simulink model "SPGF_FSK_0000_R2019b"  (R2019b)
settings: Solver=ode3  SolverName=ode4  StartTime=0.0  StopTime=1.4  FixedStep=50e-6/50  RelTol=1e-3  EnableMultiTasking=on
undefined symbols (not defined in the file): D11, Delta
libraries: powerlib x2544, powerlib_meascontrol x204, simulink x24
(part 29 of 33)

== system SPGF_FSK_0000_R2019b/W60/Pi ==
  Ground{,1..8} (9 alike) : powerlib/Elements/Ground  LConnTagsString=a
  Series RLC Branch{,1..2,27..28,33} (6 alike) : powerlib/Elements/Series RLC Branch  LConnTagsString=__new0  RConnTagsString=__new0  BranchType=RL  Resistance=R/2  Inductance=L/2  SetiL0=off  InitialCurrent=0  Capacitance=1e-6  Setx0=off  InitialVoltage=0  Measurements=None
  Series RLC Branch{10..11,13,29..30,32} (6 alike) : powerlib/Elements/Series RLC Branch  LConnTagsString=__new0  RConnTagsString=__new0  BranchType=R  Resistance=Rfg*4  Inductance=L/2  SetiL0=off  InitialCurrent=0  Capacitance=1e-6  Setx0=off  InitialVoltage=0  Measurements=None
  Series RLC Branch{9,12,14,31,40..41} (6 alike) : powerlib/Elements/Series RLC Branch  LConnTagsString=__new0  RConnTagsString=__new0  BranchType=C  Resistance=R/2  Inductance=L/2  SetiL0=off  InitialCurrent=0  Capacitance=Cfg*0.25  Setx0=off  InitialVoltage=0  Measurements=None
  Series RLC Branch15 : powerlib/Elements/Series RLC Branch  LConnTagsString=__new0  RConnTagsString=__new0  BranchType=R  Resistance=Rfg*2  Inductance=L/2  SetiL0=off  InitialCurrent=0  Capacitance=1e-6  Setx0=off  InitialVoltage=0  Measurements=None
  Series RLC Branch16 : powerlib/Elements/Series RLC Branch  LConnTagsString=__new0  RConnTagsString=__new0  BranchType=R  Resistance=Rfg*2  Inductance=L/2  SetiL0=off  InitialCurrent=0  Capacitance=1e-6  Setx0=off  InitialVoltage=0  Measurements=None
  Series RLC Branch17 : powerlib/Elements/Series RLC Branch  LConnTagsString=__new0  RConnTagsString=__new0  BranchType=C  Resistance=R/2  Inductance=L/2  SetiL0=off  InitialCurrent=0  Capacitance=Cfg*0.5  Setx0=off  InitialVoltage=0  Measurements=None
  Series RLC Branch18 : powerlib/Elements/Series RLC Branch  LConnTagsString=__new0  RConnTagsString=__new0  BranchType=R  Resistance=Rfg*2  Inductance=L/2  SetiL0=off  InitialCurrent=0  Capacitance=1e-6  Setx0=off  InitialVoltage=0  Measurements=None
  Series RLC Branch19 : powerlib/Elements/Series RLC Branch  LConnTagsString=__new0  RConnTagsString=__new0  BranchType=C  Resistance=R/2  Inductance=L/2  SetiL0=off  InitialCurrent=0  Capacitance=Cfg*0.5  Setx0=off  InitialVoltage=0  Measurements=None
  Series RLC Branch20 : powerlib/Elements/Series RLC Branch  LConnTagsString=__new0  RConnTagsString=__new0  BranchType=C  Resistance=R/2  Inductance=L/2  SetiL0=off  InitialCurrent=0  Capacitance=Cmf*0.5  Setx0=off  InitialVoltage=0  Measurements=None
  Series RLC Branch21 : powerlib/Elements/Series RLC Branch  LConnTagsString=__new0  RConnTagsString=__new0  BranchType=R  Resistance=Rmf*2  Inductance=L/2  SetiL0=off  InitialCurrent=0  Capacitance=1e-6  Setx0=off  InitialVoltage=0  Measurements=None
  Series RLC Branch22 : powerlib/Elements/Series RLC Branch  LConnTagsString=__new0  RConnTagsString=__new0  BranchType=C  Resistance=R/2  Inductance=L/2  SetiL0=off  InitialCurrent=0  Capacitance=Cmf*0.5  Setx0=off  InitialVoltage=0  Measurements=None
  Series RLC Branch23 : powerlib/Elements/Series RLC Branch  LConnTagsString=__new0  RConnTagsString=__new0  BranchType=R  Resistance=Rmf*2  Inductance=L/2  SetiL0=off  InitialCurrent=0  Capacitance=1e-6  Setx0=off  InitialVoltage=0  Measurements=None
  Series RLC Branch24 : powerlib/Elements/Series RLC Branch  LConnTagsString=__new0  RConnTagsString=__new0  BranchType=C  Resistance=R/2  Inductance=L/2  SetiL0=off  InitialCurrent=0  Capacitance=Cmf*0.5  Setx0=off  InitialVoltage=0  Measurements=None
  Series RLC Branch25 : powerlib/Elements/Series RLC Branch  LConnTagsString=__new0  RConnTagsString=__new0  BranchType=R  Resistance=Rmf*2  Inductance=L/2  SetiL0=off  InitialCurrent=0  Capacitance=1e-6  Setx0=off  InitialVoltage=0  Measurements=None
  Series RLC Branch26 : powerlib/Elements/Series RLC Branch  LConnTagsString=__new0  RConnTagsString=__new0  BranchType=C  Resistance=R/2  Inductance=L/2  SetiL0=off  InitialCurrent=0  Capacitance=Cfg*0.5  Setx0=off  InitialVoltage=0  Measurements=None
  Series RLC Branch{3,5,7,34,36,38} (6 alike) : powerlib/Elements/Series RLC Branch  LConnTagsString=__new0  RConnTagsString=__new0  BranchType=C  Resistance=R/2  Inductance=L/2  SetiL0=off  InitialCurrent=0  Capacitance=Cmf*0.25  Setx0=off  InitialVoltage=0  Measurements=None
  Series RLC Branch{4,6,8,35,37,39} (6 alike) : powerlib/Elements/Series RLC Branch  LConnTagsString=__new0  RConnTagsString=__new0  BranchType=R  Resistance=Rmf*4  Inductance=L/2  SetiL0=off  InitialCurrent=0  Capacitance=1e-6  Setx0=off  InitialVoltage=0  Measurements=None
  A : PMIOPort  Side=Left
  B : PMIOPort  Port=2  Side=Left
  C : PMIOPort  Port=3  Side=Left
  a : PMIOPort  Port=4  Side=Right
  b : PMIOPort  Port=5  Side=Right
  c : PMIOPort  Port=6  Side=Right
  connections:
  Series RLC Branch12/LConn1 -- Series RLC Branch11/LConn1 -- Series RLC Branch5/LConn1 -- Series RLC Branch6/LConn1 -- B/RConn1 -- Series RLC Branch4/RConn1 -- Series RLC Branch3/RConn1 -- Series RLC Branch1/LConn1
  Series RLC Branch13/LConn1 -- A/RConn1 -- Series RLC Branch4/LConn1 -- Series RLC Branch3/LConn1 -- Series RLC Branch7/LConn1 -- Series RLC Branch8/LConn1 -- Series RLC Branch/LConn1 -- Series RLC Branch14/LConn1
  Series RLC Branch9/LConn1 -- Series RLC Branch2/LConn1 -- Series RLC Branch8/RConn1 -- Series RLC Branch7/RConn1 -- C/RConn1 -- Series RLC Branch5/RConn1 -- Series RLC Branch6/RConn1 -- Series RLC Branch10/LConn1
  Series RLC Branch9/RConn1 -- Ground/LConn1 -- Series RLC Branch10/RConn1
  Series RLC Branch12/RConn1 -- Series RLC Branch11/RConn1 -- Ground1/LConn1
  Series RLC Branch13/RConn1 -- Series RLC Branch14/RConn1 -- Ground2/LConn1
  Series RLC Branch17/LConn1 -- Series RLC Branch16/LConn1 -- Series RLC Branch28/LConn1 -- Series RLC Branch1/RConn1 -- Series RLC Branch23/LConn1 -- Series RLC Branch22/LConn1 -- Series RLC Branch20/RConn1 -- Series RLC Branch21/RConn1
  Series RLC Branch21/LConn1 -- Series RLC Branch20/LConn1 -- Series RLC Branch/RConn1 -- Series RLC Branch27/LConn1 -- Series RLC Branch19/LConn1 -- Series RLC Branch18/LConn1 -- Series RLC Branch24/LConn1 -- Series RLC Branch25/LConn1
  Series RLC Branch26/LConn1 -- Series RLC Branch15/LConn1 -- Series RLC Branch2/RConn1 -- Series RLC Branch33/LConn1 -- Series RLC Branch25/RConn1 -- Series RLC Branch24/RConn1 -- Series RLC Branch22/RConn1 -- Series RLC Branch23/RConn1
  Series RLC Branch26/RConn1 -- Series RLC Branch15/RConn1 -- Ground3/LConn1
  Ground4/LConn1 -- Series RLC Branch17/RConn1 -- Series RLC Branch16/RConn1
  Ground5/LConn1 -- Series RLC Branch18/RConn1 -- Series RLC Branch19/RConn1
  Series RLC Branch31/LConn1 -- b/RConn1 -- Series RLC Branch35/RConn1 -- Series RLC Branch34/RConn1 -- Series RLC Branch36/LConn1 -- Series RLC Branch37/LConn1 -- Series RLC Branch28/RConn1 -- Series RLC Branch30/LConn1
  Series RLC Branch34/LConn1 -- a/RConn1 -- Series RLC Branch41/LConn1 -- Series RLC Branch32/LConn1 -- Series RLC Branch38/LConn1 -- Series RLC Branch39/LConn1 -- Series RLC Branch27/RConn1 -- Series RLC Branch35/LConn1
  Series RLC Branch29/LConn1 -- Series RLC Branch36/RConn1 -- Series RLC Branch37/RConn1 -- c/RConn1 -- Series RLC Branch39/RConn1 -- Series RLC Branch38/RConn1 -- Series RLC Branch33/RConn1 -- Series RLC Branch40/LConn1
  Series RLC Branch29/RConn1 -- Series RLC Branch40/RConn1 -- Ground6/LConn1
  Series RLC Branch31/RConn1 -- Series RLC Branch30/RConn1 -- Ground7/LConn1
  Series RLC Branch32/RConn1 -- Series RLC Branch41/RConn1 -- Ground8/LConn1

== system SPGF_FSK_0000_R2019b/W60/Q ==
  breaker : Subsystem  Commented=on  mask{SwitchA=off, SwitchB=off, SwitchC=off, InitialStatus=[1 1 1], BreakerResistance=0.0001, SnubberResistance=1e6, SnubberCapacitance=inf, TransitionTimes=[0.5 0.7], ShiftTimes=[0 0 0]}
      mask prompts: SwitchA "Switching of phase A"; SwitchB "Switching of phase B"; SwitchC "Switching of phase C"; InitialStatus "Initial status of phase breaker [A, B, C]"; BreakerResistance "Breaker resistance Ron (ohms) :"; SnubberResistance "Snubbers resistance Rp (ohms) :"; SnubberCapacitance "Snubbers capacitance Cp (F) :"; TransitionTimes "Transition times (s) :"; ShiftTimes "Time differences for switch [tA, tB, tC] (s) :"
      mask init: same as SPGF_FSK_0000_R2019b/Feed/Q/breaker
      mask Display:
      | % port_label('input',1,'Iabc');
      | 
      | port_label('lconn',1,'A');
      | port_label('lconn',2,'B');
      | port_label('lconn',3,'C');
      | 
      | port_label('rconn',1,'a');
      | port_label('rconn',2,'b');
      | port_label('rconn',3,'c');
      | 
      | disp('   Q    ');
  meas : Subsystem
  shunt : Subsystem
  A : PMIOPort  Side=Right
  B : PMIOPort  Port=2  Side=Right
  C : PMIOPort  Port=3  Side=Right
  a : PMIOPort  Port=4  Side=Left
  b : PMIOPort  Port=5  Side=Left
  c : PMIOPort  Port=6  Side=Left
  connections:
  shunt/LConn3 -- C/RConn1 -- breaker/LConn3
  shunt/LConn2 -- B/RConn1 -- breaker/LConn2
  A/RConn1 -- shunt/LConn1 -- breaker/LConn1
  meas/RConn1 -- a/RConn1
  meas/RConn2 -- b/RConn1
  meas/RConn3 -- c/RConn1
  meas/LConn3 -- breaker/RConn3 -- shunt/RConn3
  meas/LConn2 -- breaker/RConn2 -- shunt/RConn2
  meas/LConn1 -- breaker/RConn1 -- shunt/RConn1

== system SPGF_FSK_0000_R2019b/W60/concentrated ==
  Ccs/1 : powerlib/Elements/Series RLC Branch  LConnTagsString=__new0  RConnTagsString=__new0  BranchType=C  Resistance=190  Inductance=1e-3  SetiL0=off  InitialCurrent=0  Capacitance=-C_matrix(1,2)/2  Setx0=off  InitialVoltage=0  Measurements=None
  Ccs/2 : powerlib/Elements/Series RLC Branch  LConnTagsString=__new0  RConnTagsString=__new0  BranchType=C  Resistance=190  Inductance=1e-3  SetiL0=off  InitialCurrent=0  Capacitance=-C_matrix(1,2)/2  Setx0=off  InitialVoltage=0  Measurements=None
  Ccs2/1 : powerlib/Elements/Series RLC Branch  LConnTagsString=__new0  RConnTagsString=__new0  BranchType=C  Resistance=190  Inductance=1e-3  SetiL0=off  InitialCurrent=0  Capacitance=-C_matrix(3,4)/2  Setx0=off  InitialVoltage=0  Measurements=None
  Ccs2/2 : powerlib/Elements/Series RLC Branch  LConnTagsString=__new0  RConnTagsString=__new0  BranchType=C  Resistance=190  Inductance=1e-3  SetiL0=off  InitialCurrent=0  Capacitance=-C_matrix(3,4)/2  Setx0=off  InitialVoltage=0  Measurements=None
  Ccs2/3 : powerlib/Elements/Series RLC Branch  LConnTagsString=__new0  RConnTagsString=__new0  BranchType=R  Resistance=-Rg_matrix(3,4)*2  Inductance=1e-3  SetiL0=off  InitialCurrent=0  Capacitance=Rg_matrix(3,4)*2  Setx0=off  InitialVoltage=0  Measurements=None
  Ccs2/4 : powerlib/Elements/Series RLC Branch  LConnTagsString=__new0  RConnTagsString=__new0  BranchType=R  Resistance=-Rg_matrix(3,4)*2  Inductance=1e-3  SetiL0=off  InitialCurrent=0  Capacitance=Rg_matrix(3,4)*2  Setx0=off  InitialVoltage=0  Measurements=None
  Ccs3/1 : powerlib/Elements/Series RLC Branch  LConnTagsString=__new0  RConnTagsString=__new0  BranchType=C  Resistance=190  Inductance=1e-3  SetiL0=off  InitialCurrent=0  Capacitance=-C_matrix(5,6)/2  Setx0=off  InitialVoltage=0  Measurements=None
  Ccs3/2 : powerlib/Elements/Series RLC Branch  LConnTagsString=__new0  RConnTagsString=__new0  BranchType=C  Resistance=190  Inductance=1e-3  SetiL0=off  InitialCurrent=0  Capacitance=-C_matrix(5,6)/2  Setx0=off  InitialVoltage=0  Measurements=None
  Ccs3/3 : powerlib/Elements/Series RLC Branch  LConnTagsString=__new0  RConnTagsString=__new0  BranchType=R  Resistance=-Rg_matrix(5,6)*2  Inductance=1e-3  SetiL0=off  InitialCurrent=0  Capacitance=-C_matrix(5,6)/2  Setx0=off  InitialVoltage=0  Measurements=None
  Ccs3/4 : powerlib/Elements/Series RLC Branch  LConnTagsString=__new0  RConnTagsString=__new0  BranchType=R  Resistance=-Rg_matrix(5,6)*2  Inductance=1e-3  SetiL0=off  InitialCurrent=0  Capacitance=-C_matrix(5,6)/2  Setx0=off  InitialVoltage=0  Measurements=None
  Csg/2 : powerlib/Elements/Series RLC Branch  LConnTagsString=__new0  RConnTagsString=__new0  BranchType=C  Resistance=190  Inductance=1e-3  SetiL0=off  InitialCurrent=0  Capacitance=( C_matrix(1,2) + C_matrix(2,2) )/2  Setx0=off  InitialVoltage=0  Measurements=None
  Csg1/1 : powerlib/Elements/Series RLC Branch  LConnTagsString=__new0  RConnTagsString=__new0  BranchType=C  Resistance=190  Inductance=1e-3  SetiL0=off  InitialCurrent=0  Capacitance=( C_matrix(1,2) + C_matrix(2,2) )/2  Setx0=off  InitialVoltage=0  Measurements=None
  Csg2/1 : powerlib/Elements/Series RLC Branch  LConnTagsString=__new0  RConnTagsString=__new0  BranchType=C  Resistance=190  Inductance=1e-3  SetiL0=off  InitialCurrent=0  Capacitance=( C_matrix(3,4) + C_matrix(4,4) )/2  Setx0=off  InitialVoltage=0  Measurements=None
  Csg2/2 : powerlib/Elements/Series RLC Branch  LConnTagsString=__new0  RConnTagsString=__new0  BranchType=C  Resistance=190  Inductance=1e-3  SetiL0=off  InitialCurrent=0  Capacitance=( C_matrix(3,4) + C_matrix(4,4) )/2  Setx0=off  InitialVoltage=0  Measurements=None
  Csg3/1 : powerlib/Elements/Series RLC Branch  LConnTagsString=__new0  RConnTagsString=__new0  BranchType=C  Resistance=190  Inductance=1e-3  SetiL0=off  InitialCurrent=0  Capacitance=( C_matrix(5,6) + C_matrix(6,6) ) /2  Setx0=off  InitialVoltage=0  Measurements=None
  Csg3/2 : powerlib/Elements/Series RLC Branch  LConnTagsString=__new0  RConnTagsString=__new0  BranchType=C  Resistance=190  Inductance=1e-3  SetiL0=off  InitialCurrent=0  Capacitance=( C_matrix(5,6) + C_matrix(6,6) ) /2  Setx0=off  InitialVoltage=0  Measurements=None
  Ground{1..4} (4 alike) : powerlib/Elements/Ground  LConnTagsString=a
  RL : powerlib/Elements/Mutual Inductance  LConnTagsString=a|b|c|L4|L5|L6  RConnTagsString=A|B|C|R4|R5|R6  TypeOfMutual=Generalized mutual inductance  NumberOfWindings=6  SelfImpedance1=[1.1 1.1e-03]  SelfImpedance2=[ 1.1 1.1e-03]  ThreeWindings=on  SelfImpedance3=[ 1.1 1.1e-03]  MutualImpedance=[1.0 1.0e-03]  InductanceMatrix=L_matrix  ResistanceMatrix=R_matrix  Measurements=None
      settings: AttributesFormatString=\n
  Rcs*2 : powerlib/Elements/Series RLC Branch  LConnTagsString=__new0  RConnTagsString=__new0  BranchType=R  Resistance=-Rg_matrix(1,2)*2  Inductance=1e-3  SetiL0=off  InitialCurrent=0  Capacitance=Rg_matrix(1,2)*2  Setx0=off  InitialVoltage=0  Measurements=None
  Rgcs1/1 : powerlib/Elements/Series RLC Branch  LConnTagsString=__new0  RConnTagsString=__new0  BranchType=R  Resistance=-Rg_matrix(1,2)*2  Inductance=1e-3  SetiL0=off  InitialCurrent=0  Capacitance=Rg_matrix(1,2)*2  Setx0=off  InitialVoltage=0  Measurements=None
  Rgsg1/1 : powerlib/Elements/Series RLC Branch  LConnTagsString=__new0  RConnTagsString=__new0  BranchType=R  Resistance=(Rg_matrix(4,4)+Rg_matrix(3,4))*2  Inductance=1e-3  SetiL0=off  InitialCurrent=0  Capacitance=Rg_matrix(1,2)*2  Setx0=off  InitialVoltage=0  Measurements=None
  Rgsg1/2 : powerlib/Elements/Series RLC Branch  LConnTagsString=__new0  RConnTagsString=__new0  BranchType=R  Resistance=(Rg_matrix(2,2)+Rg_matrix(1,2))*2  Inductance=1e-3  SetiL0=off  InitialCurrent=0  Capacitance=Rg_matrix(1,2)*2  Setx0=off  InitialVoltage=0  Measurements=None
  Rgsg1/3 : powerlib/Elements/Series RLC Branch  LConnTagsString=__new0  RConnTagsString=__new0  BranchType=R  Resistance=(Rg_matrix(4,4)+Rg_matrix(3,4))*2  Inductance=1e-3  SetiL0=off  InitialCurrent=0  Capacitance=Rg_matrix(1,2)*2  Setx0=off  InitialVoltage=0  Measurements=None
  Rgsg1/4 : powerlib/Elements/Series RLC Branch  LConnTagsString=__new0  RConnTagsString=__new0  BranchType=R  Resistance=(Rg_matrix(2,2)+Rg_matrix(1,2))*2  Inductance=1e-3  SetiL0=off  InitialCurrent=0  Capacitance=Rg_matrix(1,2)*2  Setx0=off  InitialVoltage=0  Measurements=None
  Rsg*2 : powerlib/Elements/Series RLC Branch  LConnTagsString=__new0  RConnTagsString=__new0  BranchType=R  Resistance=(Rg_matrix(6,6)+Rg_matrix(5,6))*2  Inductance=1e-3  SetiL0=off  InitialCurrent=0  Capacitance=Rg_matrix(1,2)*2  Setx0=off  InitialVoltage=0  Measurements=None
  Rsg1/1 : powerlib/Elements/Series RLC Branch  LConnTagsString=__new0  RConnTagsString=__new0  BranchType=R  Resistance=(Rg_matrix(6,6)+Rg_matrix(5,6))*2  Inductance=1e-3  SetiL0=off  InitialCurrent=0  Capacitance=Rg_matrix(1,2)*2  Setx0=off  InitialVoltage=0  Measurements=None
  A : PMIOPort  Side=Left
  B : PMIOPort  Port=2  Side=Left
  C : PMIOPort  Port=3  Side=Left
  a : PMIOPort  Port=4  Side=Right
  b : PMIOPort  Port=5  Side=Right
  c : PMIOPort  Port=6  Side=Right
  connections:
  RL/LConn6 -- Ground3/LConn1 -- Rgsg1/2/LConn1 -- Csg/2/LConn1 -- Rcs*2/LConn1 -- Ccs/2/LConn1 -- RL/LConn2 -- RL/LConn4 -- Rgsg1/1/LConn1 -- Csg2/2/LConn1 -- Ccs2/3/LConn1 -- Ccs2/2/LConn1 -- Rsg*2/LConn1 -- Csg3/2/LConn1 -- Ccs3/3/LConn1 -- Ccs3/2/LConn1
  Rsg1/1/RConn1 -- Rgsg1/3/RConn1 -- Rgsg1/4/RConn1 -- Csg3/1/RConn1 -- Csg2/1/RConn1 -- Ground2/LConn1 -- Csg1/1/RConn1
  Rgsg1/3/LConn1 -- Ccs2/4/LConn1 -- Csg2/1/LConn1 -- Ccs2/1/LConn1 -- RL/RConn4 -- Rgsg1/4/LConn1 -- Rgcs1/1/LConn1 -- Csg1/1/LConn1 -- Ccs/1/LConn1 -- RL/RConn2 -- Ground4/LConn1 -- RL/RConn6 -- Ccs3/1/LConn1 -- Rsg1/1/LConn1 -- Ccs3/4/LConn1 -- Csg3/1/LConn1
  Rsg*2/RConn1 -- Rgsg1/1/RConn1 -- Rgsg1/2/RConn1 -- Csg3/2/RConn1 -- Csg2/2/RConn1 -- Ground1/LConn1 -- Csg/2/RConn1
  a/RConn1 -- RL/RConn1 -- Rgcs1/1/RConn1 -- Ccs/1/RConn1
  b/RConn1 -- RL/RConn3 -- Ccs2/4/RConn1 -- Ccs2/1/RConn1
  Ccs3/1/RConn1 -- c/RConn1 -- RL/RConn5 -- Ccs3/4/RConn1
  RL/LConn1 -- A/RConn1 -- Rcs*2/RConn1 -- Ccs/2/RConn1
  RL/LConn3 -- B/RConn1 -- Ccs2/3/RConn1 -- Ccs2/2/RConn1
  Ccs3/2/RConn1 -- C/RConn1 -- RL/LConn5 -- Ccs3/3/RConn1

== system SPGF_FSK_0000_R2019b/W61/Q ==
  breaker : Subsystem  Commented=on  mask{SwitchA=off, SwitchB=off, SwitchC=off, InitialStatus=[1 1 1], BreakerResistance=0.0001, SnubberResistance=1e6, SnubberCapacitance=inf, TransitionTimes=[0.5 0.7], ShiftTimes=[0 0 0]}
      mask prompts: SwitchA "Switching of phase A"; SwitchB "Switching of phase B"; SwitchC "Switching of phase C"; InitialStatus "Initial status of phase breaker [A, B, C]"; BreakerResistance "Breaker resistance Ron (ohms) :"; SnubberResistance "Snubbers resistance Rp (ohms) :"; SnubberCapacitance "Snubbers capacitance Cp (F) :"; TransitionTimes "Transition times (s) :"; ShiftTimes "Time differences for switch [tA, tB, tC] (s) :"
      mask init: same as SPGF_FSK_0000_R2019b/Feed/Q/breaker
      mask Display:
      | % port_label('input',1,'Iabc');
      | 
      | port_label('lconn',1,'A');
      | port_label('lconn',2,'B');
      | port_label('lconn',3,'C');
      | 
      | port_label('rconn',1,'a');
      | port_label('rconn',2,'b');
      | port_label('rconn',3,'c');
      | 
      | disp('   Q    ');
  meas : Subsystem
  shunt : Subsystem
  A : PMIOPort  Side=Right
  B : PMIOPort  Port=2  Side=Right
  C : PMIOPort  Port=3  Side=Right
  a : PMIOPort  Port=4  Side=Left
  b : PMIOPort  Port=5  Side=Left
  c : PMIOPort  Port=6  Side=Left
  connections:
  shunt/RConn1 -- breaker/RConn1 -- meas/LConn1
  shunt/RConn2 -- breaker/RConn2 -- meas/LConn2
  shunt/RConn3 -- breaker/RConn3 -- meas/LConn3
  meas/RConn3 -- c/RConn1
  meas/RConn2 -- b/RConn1
  meas/RConn1 -- a/RConn1
  breaker/LConn1 -- shunt/LConn1 -- A/RConn1
  breaker/LConn2 -- B/RConn1 -- shunt/LConn2
  breaker/LConn3 -- C/RConn1 -- shunt/LConn3

== system SPGF_FSK_0000_R2019b/measurements/Fourier Block abc ==
  abc : Inport
  Demux1 : Demux  Commented=on  Outputs=9
  Scope13 : Scope
  Sequence Analyzer9 : powerlib_meascontrol/Measurements/Sequence Analyzer  Freq=50  n=17  seq=Positive  InInit=[0, 0]  Ts=FTime
  Terminator9 : Terminator
  wires:
  abc/1 -> Sequence Analyzer9/1
  Sequence Analyzer9/2 -> Terminator9/1
  Sequence Analyzer9/1 -> Scope13/1, Demux1/1

== system SPGF_FSK_0000_R2019b/measurements/Fourier Block u ==
  u : Inport
  Demux1 : Demux  Commented=on  Outputs=9
  Fourier10 : powerlib_meascontrol/Measurements/Fourier  Freq=50  n=[1 2 3 5 7 9 11 13 17]  InInit=[0, 0]  Ts=FTime
  Scope13 : Scope
  Terminator10 : Terminator
  wires:
  u/1 -> Fourier10/1
  Fourier10/1 -> Demux1/1, Scope13/1
  Fourier10/2 -> Terminator10/1

== system SPGF_FSK_0000_R2019b/measurements/PQ1 ==
  Vmag_seq : Inport
  Vang : Inport  Port=2
  Imag_seq : Inport  Port=3
  Iang : Inport  Port=4
  Deg->Rad : Gain  Gain=pi/180  SaturateOnIntegerOverflow=on  OutDataTypeStr=Inherit: Same as input  ParamDataTypeStr=Inherit: Same as input
  Gain1 : Gain  Gain=3/2  SaturateOnIntegerOverflow=on  OutDataTypeStr=Inherit: Same as input  ParamDataTypeStr=Inherit: Same as input
  Product : Product  InputSameDT=on  SaturateOnIntegerOverflow=on  OutDataTypeStr=Inherit: Same as first input
  Product1 : Product  InputSameDT=on  SaturateOnIntegerOverflow=on  OutDataTypeStr=Inherit: Same as first input
  Product3 : Product  InputSameDT=on  SaturateOnIntegerOverflow=on  OutDataTypeStr=Inherit: Same as first input
  Sum : Sum  Inputs=+-  InputSameDT=on  SaturateOnIntegerOverflow=on  OutDataTypeStr=Inherit: Same as first input
  Trigonometric Function1 : Trigonometry  Operator=cos
  Trigonometric Function2 : Trigonometry
  P : Outport
  Q : Outport  Port=2
  wires:
  Trigonometric Function1/1 -> Product1/2
  Sum/1 -> Deg->Rad/1
  Imag_seq/1 -> Product/2
  Product/1 -> Gain1/1  "V1 *I1"
  Trigonometric Function2/1 -> Product3/2
  Gain1/1 -> Product1/1, Product3/1
  Vmag_seq/1 -> Product/1
  Deg->Rad/1 -> Trigonometric Function2/1, Trigonometric Function1/1  "phi"
  Product3/1 -> Q/1
  Iang/1 -> Sum/2
  Vang/1 -> Sum/1
  Product1/1 -> P/1

== system SPGF_FSK_0000_R2019b/measurements/PQ8 ==
  Vmag_seq : Inport
  Vang : Inport  Port=2
  Imag_seq : Inport  Port=3
  Iang : Inport  Port=4
  Deg->Rad : Gain  Gain=pi/180  SaturateOnIntegerOverflow=on  OutDataTypeStr=Inherit: Same as input  ParamDataTypeStr=Inherit: Same as input
  Gain1 : Gain  Gain=3/2  SaturateOnIntegerOverflow=on  OutDataTypeStr=Inherit: Same as input  ParamDataTypeStr=Inherit: Same as input
  Product : Product  InputSameDT=on  SaturateOnIntegerOverflow=on  OutDataTypeStr=Inherit: Same as first input
  Product1 : Product  InputSameDT=on  SaturateOnIntegerOverflow=on  OutDataTypeStr=Inherit: Same as first input
  Product3 : Product  InputSameDT=on  SaturateOnIntegerOverflow=on  OutDataTypeStr=Inherit: Same as first input
  Sum : Sum  Inputs=+-  InputSameDT=on  SaturateOnIntegerOverflow=on  OutDataTypeStr=Inherit: Same as first input
  Trigonometric Function1 : Trigonometry  Operator=cos
  Trigonometric Function2 : Trigonometry
  P : Outport
  Q : Outport  Port=2
  wires:
  Product1/1 -> P/1
  Vang/1 -> Sum/1
  Iang/1 -> Sum/2
  Product3/1 -> Q/1
  Deg->Rad/1 -> Trigonometric Function1/1, Trigonometric Function2/1  "phi"
  Vmag_seq/1 -> Product/1
  Gain1/1 -> Product3/1, Product1/1
  Trigonometric Function2/1 -> Product3/2
  Product/1 -> Gain1/1  "V1 *I1"
  Imag_seq/1 -> Product/2
  Sum/1 -> Deg->Rad/1
  Trigonometric Function1/1 -> Product1/2

== system SPGF_FSK_0000_R2019b/measurements/RMS1 ==
  abc : Inport
  Gain25 : Gain  Gain=1/sqrt(2)
  Rate Transition : RateTransition
  Rate Transition1 : RateTransition
  Sequence Analyzer : powerlib_meascontrol/Measurements/Sequence Analyzer  Freq=50  n=1  seq=Positive  InInit=[1, 0]  Ts=FTime
  Terminator19 : Terminator
  I1 : Outport
  wires:
  Sequence Analyzer/2 -> Terminator19/1
  Gain25/1 -> Rate Transition1/1
  Sequence Analyzer/1 -> Gain25/1
  abc/1 -> Rate Transition/1
  Rate Transition/1 -> Sequence Analyzer/1
  Rate Transition1/1 -> I1/1

== system SPGF_FSK_0000_R2019b/measurements/RMS10 ==
  i : Inport
  Fourier36 : powerlib_meascontrol/Measurements/Fourier  Freq=50  n=1  InInit=[0, 0]  Ts=FTime
  Gain25 : Gain  Gain=1/sqrt(2)
  Rate Transition : RateTransition
  Rate Transition1 : RateTransition
  Terminator19 : Terminator
  I : Outport
  wires:
  Rate Transition1/1 -> I/1
  Rate Transition/1 -> Fourier36/1
  Fourier36/2 -> Terminator19/1
  Gain25/1 -> Rate Transition1/1
  Fourier36/1 -> Gain25/1
  i/1 -> Rate Transition/1

== system SPGF_FSK_0000_R2019b/measurements/RMS11 ==
  i : Inport
  Fourier36 : powerlib_meascontrol/Measurements/Fourier  Freq=50  n=1  InInit=[0, 0]  Ts=FTime
  Gain25 : Gain  Gain=1/sqrt(2)
  Rate Transition : RateTransition
  Rate Transition1 : RateTransition
  Terminator19 : Terminator
  I : Outport
  wires:
  i/1 -> Rate Transition/1
  Fourier36/1 -> Gain25/1
  Gain25/1 -> Rate Transition1/1
  Fourier36/2 -> Terminator19/1
  Rate Transition/1 -> Fourier36/1
  Rate Transition1/1 -> I/1

== system SPGF_FSK_0000_R2019b/measurements/RMS12 ==
  abc : Inport
  Gain25 : Gain  Gain=1/sqrt(2)
  Rate Transition : RateTransition
  Rate Transition1 : RateTransition
  Sequence Analyzer : powerlib_meascontrol/Measurements/Sequence Analyzer  Freq=50  n=1  seq=Positive  InInit=[1, 0]  Ts=FTime
  Terminator19 : Terminator
  I1 : Outport
  wires:
  Sequence Analyzer/2 -> Terminator19/1
  Gain25/1 -> Rate Transition1/1
  Sequence Analyzer/1 -> Gain25/1
  abc/1 -> Rate Transition/1
  Rate Transition/1 -> Sequence Analyzer/1
  Rate Transition1/1 -> I1/1

== system SPGF_FSK_0000_R2019b/measurements/RMS13 ==
  i : Inport
  Fourier36 : powerlib_meascontrol/Measurements/Fourier  Freq=50  n=1  InInit=[0, 0]  Ts=FTime
  Gain25 : Gain  Gain=1/sqrt(2)
  Rate Transition : RateTransition
  Rate Transition1 : RateTransition
  Terminator19 : Terminator
  I : Outport
  wires:
  Rate Transition1/1 -> I/1
  Rate Transition/1 -> Fourier36/1
  Fourier36/2 -> Terminator19/1
  Gain25/1 -> Rate Transition1/1
  Fourier36/1 -> Gain25/1
  i/1 -> Rate Transition/1

== system SPGF_FSK_0000_R2019b/measurements/RMS14 ==
  abc : Inport
  Gain25 : Gain  Gain=1/sqrt(2)
  Rate Transition : RateTransition
  Rate Transition1 : RateTransition
  Sequence Analyzer : powerlib_meascontrol/Measurements/Sequence Analyzer  Freq=50  n=1  seq=Positive  InInit=[1, 0]  Ts=FTime
  Terminator19 : Terminator
  I1 : Outport
  wires:
  Rate Transition1/1 -> I1/1
  Rate Transition/1 -> Sequence Analyzer/1
  abc/1 -> Rate Transition/1
  Sequence Analyzer/1 -> Gain25/1
  Gain25/1 -> Rate Transition1/1
  Sequence Analyzer/2 -> Terminator19/1

== system SPGF_FSK_0000_R2019b/measurements/RMS2 ==
  i : Inport
  Fourier36 : powerlib_meascontrol/Measurements/Fourier  Freq=50  n=1  InInit=[0, 0]  Ts=FTime
  Gain25 : Gain  Gain=1/sqrt(2)
  Rate Transition : RateTransition
  Rate Transition1 : RateTransition
  Terminator19 : Terminator
  I : Outport
  wires:
  i/1 -> Rate Transition/1
  Fourier36/1 -> Gain25/1
  Gain25/1 -> Rate Transition1/1
  Fourier36/2 -> Terminator19/1
  Rate Transition/1 -> Fourier36/1
  Rate Transition1/1 -> I/1

== system SPGF_FSK_0000_R2019b/measurements/RMS3 ==
  abc : Inport
  Gain25 : Gain  Gain=1/sqrt(2)
  Rate Transition : RateTransition
  Rate Transition1 : RateTransition
  Sequence Analyzer : powerlib_meascontrol/Measurements/Sequence Analyzer  Freq=50  n=1  seq=Positive  InInit=[1, 0]  Ts=FTime
  Terminator19 : Terminator
  I1 : Outport
  wires:
  Rate Transition1/1 -> I1/1
  Rate Transition/1 -> Sequence Analyzer/1
  abc/1 -> Rate Transition/1
  Sequence Analyzer/1 -> Gain25/1
  Gain25/1 -> Rate Transition1/1
  Sequence Analyzer/2 -> Terminator19/1

== system SPGF_FSK_0000_R2019b/measurements/RMS36 ==
  abc : Inport
  Gain25 : Gain  Gain=1/sqrt(2)
  Sequence Analyzer : powerlib_meascontrol/Measurements/Sequence Analyzer  Freq=50  n=1  seq=Positive  InInit=[1, 0]  Ts=FTime
  Terminator19 : Terminator
  I1 : Outport
  wires:
  abc/1 -> Sequence Analyzer/1
  Sequence Analyzer/1 -> Gain25/1
  Gain25/1 -> I1/1
  Sequence Analyzer/2 -> Terminator19/1

== system SPGF_FSK_0000_R2019b/measurements/RMS4 ==
  i : Inport
  Fourier36 : powerlib_meascontrol/Measurements/Fourier  Freq=50  n=1  InInit=[0, 0]  Ts=FTime
  Gain25 : Gain  Gain=1/sqrt(2)
  Rate Transition : RateTransition
  Rate Transition1 : RateTransition
  Terminator19 : Terminator
  I : Outport
  wires:
  Rate Transition1/1 -> I/1
  Rate Transition/1 -> Fourier36/1
  Fourier36/2 -> Terminator19/1
  Gain25/1 -> Rate Transition1/1
  Fourier36/1 -> Gain25/1
  i/1 -> Rate Transition/1

== system SPGF_FSK_0000_R2019b/measurements/RMS44 ==
  abc : Inport
  Gain25 : Gain  Gain=1/sqrt(2)
  Sequence Analyzer : powerlib_meascontrol/Measurements/Sequence Analyzer  Freq=50  n=1  seq=Positive  InInit=[1, 0]  Ts=FTime
  Terminator19 : Terminator
  I1 : Outport
  wires:
  Sequence Analyzer/2 -> Terminator19/1
  Gain25/1 -> I1/1
  Sequence Analyzer/1 -> Gain25/1
  abc/1 -> Sequence Analyzer/1

== system SPGF_FSK_0000_R2019b/measurements/RMS45 ==
  abc : Inport
  Gain25 : Gain  Gain=1/sqrt(2)
  Sequence Analyzer : powerlib_meascontrol/Measurements/Sequence Analyzer  Freq=50  n=1  seq=Positive  InInit=[1, 0]  Ts=FTime
  Terminator19 : Terminator
  I1 : Outport
  wires:
  abc/1 -> Sequence Analyzer/1
  Sequence Analyzer/1 -> Gain25/1
  Gain25/1 -> I1/1
  Sequence Analyzer/2 -> Terminator19/1

== system SPGF_FSK_0000_R2019b/measurements/RMS46 ==
  i : Inport
  Fourier36 : powerlib_meascontrol/Measurements/Fourier  Freq=50  n=1  InInit=[0, 0]  Ts=FTime
  Gain25 : Gain  Gain=1/sqrt(2)
  Terminator19 : Terminator
  I : Outport
  wires:
  Fourier36/2 -> Terminator19/1
  Gain25/1 -> I/1
  Fourier36/1 -> Gain25/1
  i/1 -> Fourier36/1

== system SPGF_FSK_0000_R2019b/measurements/RMS5 ==
  abc : Inport
  Gain25 : Gain  Gain=1/sqrt(2)
  Rate Transition : RateTransition
  Rate Transition1 : RateTransition
  Sequence Analyzer : powerlib_meascontrol/Measurements/Sequence Analyzer  Freq=50  n=1  seq=Positive  InInit=[1, 0]  Ts=FTime
  Terminator19 : Terminator
  I1 : Outport
  wires:
  Rate Transition1/1 -> I1/1
  Rate Transition/1 -> Sequence Analyzer/1
  abc/1 -> Rate Transition/1
  Sequence Analyzer/1 -> Gain25/1
  Gain25/1 -> Rate Transition1/1
  Sequence Analyzer/2 -> Terminator19/1

== system SPGF_FSK_0000_R2019b/measurements/RMS6 ==
  i : Inport
  Fourier36 : powerlib_meascontrol/Measurements/Fourier  Freq=50  n=1  InInit=[0, 0]  Ts=FTime
  Gain25 : Gain  Gain=1/sqrt(2)
  Rate Transition : RateTransition
  Rate Transition1 : RateTransition
  Terminator19 : Terminator
  I : Outport
  wires:
  Rate Transition1/1 -> I/1
  Rate Transition/1 -> Fourier36/1
  Fourier36/2 -> Terminator19/1
  Gain25/1 -> Rate Transition1/1
  Fourier36/1 -> Gain25/1
  i/1 -> Rate Transition/1

== system SPGF_FSK_0000_R2019b/measurements/RMS7 ==
  abc : Inport
  Gain25 : Gain  Gain=1/sqrt(2)
  Rate Transition : RateTransition
  Rate Transition1 : RateTransition
  Sequence Analyzer : powerlib_meascontrol/Measurements/Sequence Analyzer  Freq=50  n=1  seq=Positive  InInit=[1, 0]  Ts=FTime
  Terminator19 : Terminator
  I1 : Outport
  wires:
  Sequence Analyzer/2 -> Terminator19/1
  Gain25/1 -> Rate Transition1/1
  Sequence Analyzer/1 -> Gain25/1
  abc/1 -> Rate Transition/1
  Rate Transition/1 -> Sequence Analyzer/1
  Rate Transition1/1 -> I1/1

== system SPGF_FSK_0000_R2019b/measurements/RMS8 ==
  i : Inport
  Fourier36 : powerlib_meascontrol/Measurements/Fourier  Freq=50  n=1  InInit=[0, 0]  Ts=FTime
  Gain25 : Gain  Gain=1/sqrt(2)
  Rate Transition : RateTransition
  Rate Transition1 : RateTransition
  Terminator19 : Terminator
  I : Outport
  wires:
  i/1 -> Rate Transition/1
  Fourier36/1 -> Gain25/1
  Gain25/1 -> Rate Transition1/1
  Fourier36/2 -> Terminator19/1
  Rate Transition/1 -> Fourier36/1
  Rate Transition1/1 -> I/1

== system SPGF_FSK_0000_R2019b/measurements/RMS9 ==
  abc : Inport
  Gain25 : Gain  Gain=1/sqrt(2)
  Rate Transition : RateTransition
  Rate Transition1 : RateTransition
  Sequence Analyzer : powerlib_meascontrol/Measurements/Sequence Analyzer  Freq=50  n=1  seq=Positive  InInit=[1, 0]  Ts=FTime
  Terminator19 : Terminator
  I1 : Outport
  wires:
  Rate Transition1/1 -> I1/1
  Rate Transition/1 -> Sequence Analyzer/1
  abc/1 -> Rate Transition/1
  Sequence Analyzer/1 -> Gain25/1
  Gain25/1 -> Rate Transition1/1
  Sequence Analyzer/2 -> Terminator19/1

== system SPGF_FSK_0000_R2019b/measurements/RXZ1 ==
  Vmag_seq : Inport
  Vang : Inport  Port=2
  Imag_seq : Inport  Port=3
  Iang : Inport  Port=4
  Add : Sum  Inputs=+-
  Divide : Product  Inputs=*/
  Gain : Gain  Gain=pi/180
  Product : Product
  Product1 : Product
  Trigonometric Function : Trigonometry
  Trigonometric Function1 : Trigonometry  Operator=cos
  R : Outport
  X : Outport  Port=2
  Z : Outport  Port=3
  Zang : Outport  Port=4
  wires:
  Iang/1 -> Add/2
  Trigonometric Function/1 -> Product1/2
  Trigonometric Function1/1 -> Product/2
  Vang/1 -> Add/1
  Divide/1 -> Z/1, Product/1, Product1/1
  Product1/1 -> X/1
  Product/1 -> R/1
  Imag_seq/1 -> Divide/2
  Vmag_seq/1 -> Divide/1
  Gain/1 -> Trigonometric Function/1, Trigonometric Function1/1
  Add/1 -> Zang/1, Gain/1

== system SPGF_FSK_0000_R2019b/measurements/RXZ7 ==
  Vmag_seq : Inport
  Vang : Inport  Port=2
  Imag_seq : Inport  Port=3
  Iang : Inport  Port=4
  Add : Sum  Inputs=+-
  Divide : Product  Inputs=*/
  Gain : Gain  Gain=pi/180
  Product : Product
  Product1 : Product
  Trigonometric Function : Trigonometry
  Trigonometric Function1 : Trigonometry  Operator=cos
  R : Outport
  X : Outport  Port=2
  Z : Outport  Port=3
  Zang : Outport  Port=4
  wires:
  Add/1 -> Gain/1, Zang/1
  Gain/1 -> Trigonometric Function1/1, Trigonometric Function/1
  Vmag_seq/1 -> Divide/1
  Imag_seq/1 -> Divide/2
  Product/1 -> R/1
  Product1/1 -> X/1
  Divide/1 -> Product1/1, Product/1, Z/1
  Vang/1 -> Add/1
  Trigonometric Function1/1 -> Product/2
  Trigonometric Function/1 -> Product1/2
  Iang/1 -> Add/2

== system SPGF_FSK_0000_R2019b/Feed/Q/breaker ==
  Fault A2 : Constant  Value=InitialStatus(3)
  Fault A3 : Constant  Value=InitialStatus(2)
  Fault A4 : Constant  Value=InitialStatus(1)
  Fault C1 : Constant  Value=SwitchC
  Fault C2 : Constant  Value=SwitchB
  Fault C3 : Constant  Value=SwitchA
  Ideal Switch A : powerlib/Power Electronics/Ideal Switch  Ron=BreakerResistance  Lon=0  IC=InitialStatus(1)  Rs=SnubberResistance  Cs=SnubberCapacitance  Measurements=off
  Ideal Switch B : powerlib/Power Electronics/Ideal Switch  Ron=BreakerResistance  Lon=0  IC=InitialStatus(2)  Rs=SnubberResistance  Cs=SnubberCapacitance  Measurements=off
  Ideal Switch C : powerlib/Power Electronics/Ideal Switch  Ron=BreakerResistance  Lon=0  IC=InitialStatus(3)  Rs=SnubberResistance  Cs=SnubberCapacitance  Measurements=off
  Stair Generator A : powerlib_meascontrol/Pulse & Signal Generators/Stair Generator  t=SwitchTimesA  e=SwitchStatusA  Ts=0
  Stair Generator B : powerlib_meascontrol/Pulse & Signal Generators/Stair Generator  t=SwitchTimesB  e=SwitchStatusB  Ts=0
  Stair Generator C : powerlib_meascontrol/Pulse & Signal Generators/Stair Generator  t=SwitchTimesB  e=SwitchStatusB  Ts=0
  Switch2 : Switch  Criteria=u2 > Threshold  Threshold=0.5
  Switch3 : Switch  Criteria=u2 > Threshold  Threshold=0.5
  Switch4 : Switch  Criteria=u2 > Threshold  Threshold=0.5
  A : PMIOPort  Side=Left
  B : PMIOPort  Port=2  Side=Left
  C : PMIOPort  Port=3  Side=Left
  a : PMIOPort  Port=4  Side=Right
  b : PMIOPort  Port=5  Side=Right
  c : PMIOPort  Port=6  Side=Right
  wires:
  Switch2/1 -> Ideal Switch C/1
  Fault A2/1 -> Switch2/3
  Fault C1/1 -> Switch2/2
  Switch3/1 -> Ideal Switch B/1
  Fault A3/1 -> Switch3/3
  Fault C2/1 -> Switch3/2
  Fault A4/1 -> Switch4/3
  Fault C3/1 -> Switch4/2
  Switch4/1 -> Ideal Switch A/1
  Stair Generator B/1 -> Switch3/1
  Stair Generator A/1 -> Switch4/1
  Stair Generator C/1 -> Switch2/1
  connections:
  Ideal Switch B/LConn1 -- B/RConn1
  Ideal Switch A/LConn1 -- A/RConn1
  Ideal Switch C/LConn1 -- C/RConn1
  Ideal Switch A/RConn1 -- a/RConn1
  b/RConn1 -- Ideal Switch B/RConn1
  c/RConn1 -- Ideal Switch C/RConn1

== system SPGF_FSK_0000_R2019b/Feed/Q/meas ==
  Add : Sum  Inputs=+++
  GainI : Gain
  GainI0 : Gain
  I A: : powerlib/Measurements/Current Measurement  PhasorSimulation=off  OutputType=Complex  PSBequivalent=0
  I B: : powerlib/Measurements/Current Measurement  PhasorSimulation=off  OutputType=Complex  PSBequivalent=0
  I C: : powerlib/Measurements/Current Measurement  PhasorSimulation=off  OutputType=Complex  PSBequivalent=0
  Mux : Mux  Inputs=3
  A : PMIOPort  Side=Left
  B : PMIOPort  Port=2  Side=Left
  C : PMIOPort  Port=3  Side=Left
  a : PMIOPort  Port=4  Side=Right
  b : PMIOPort  Port=5  Side=Right
  c : PMIOPort  Port=6  Side=Right
  tag scope: CT3I0_F=global, CTIabc_F=global
  wires:
  Mux/1 -> GainI/1
  GainI0/1 -> [CT3I0_F]
  Add/1 -> GainI0/1
  I C:/1 -> Add/3, Mux/3
  I B:/1 -> Add/2, Mux/2
  I A:/1 -> Add/1, Mux/1
  GainI/1 -> [CTIabc_F]
  connections:
  I B:/LConn1 -- B/RConn1
  I C:/LConn1 -- C/RConn1
  I A:/LConn1 -- A/RConn1
  a/RConn1 -- I A:/RConn1
  I B:/RConn1 -- b/RConn1
  I C:/RConn1 -- c/RConn1

== system SPGF_FSK_0000_R2019b/Feed/Q/shunt ==
  A : PMIOPort  Side=Left
  B : PMIOPort  Port=2  Side=Left
  C : PMIOPort  Port=3  Side=Left
  a : PMIOPort  Port=4  Side=Right
  b : PMIOPort  Port=5  Side=Right
  c : PMIOPort  Port=6  Side=Right
  connections:
  C/RConn1 -- c/RConn1
  B/RConn1 -- b/RConn1
  A/RConn1 -- a/RConn1

== system SPGF_FSK_0000_R2019b/K1/fault/Arcing ==
  I : Inport
  Enable : EnablePort  StatesWhenEnabling=reset
  Abs3 : Abs
  Add3 : Sum
  Clock : Clock
  Compare To Zero : simulink/Logic and Bit Operations/Compare To Zero  relop=~=  OutDataTypeStr=boolean
  Constant1 : Constant  Value=TheoryOfArc
  Constant4 : Constant  Value=TheoryOfArc
  DTC_B : DataTypeConversion  OutDataTypeStr=boolean
  DTC_D : DataTypeConversion  OutDataTypeStr=double
  DTC_D1 : DataTypeConversion  OutDataTypeStr=double
  Demux : Demux  Outputs=2
  Fault A10 : Constant
  Fault A11 : Constant  Value=0
  Fault A13 : Constant
  Fault A14 : Constant  Value=0
  Hit Crossing : HitCross
  Memory : Memory
  Product : Product
  Product1 : Product
  R-S Flip-Flop : Subsystem  mask(RSFlipFlop){InitialCondition=0}
      mask prompts: InitialCondition "Initial condition (state of Q)"
      mask help: R-S Flip-Flop Block
  Ramp : simulink/Sources/Ramp  slope=Slope  start=BeginFaultTime  InitialOutput=ArcingVoltage(1)
  Relational Operator4 : RelationalOperator  OutDataTypeStr=boolean  RndMeth=Nearest
  Relational Operator5 : RelationalOperator  OutDataTypeStr=boolean  RndMeth=Nearest
  SW_1 : MultiPortSwitch  DataPortForDefault=Additional data port
  SW_2 : Switch  Criteria=u2 > Threshold  Threshold=2
  Switch4 : Switch  Criteria=u2 > Threshold  Threshold=0.5
  Terminator3 : Terminator
  TimeDiff : Constant  Value=.015
  Triggered Subsystem1 : Subsystem  TreatAsAtomicUnit=on
  O : Outport  InitialOutput=[0]
  wires:
  Memory/1 -> Triggered Subsystem1/Trigger
  Constant1/1 -> SW_1/1
  SW_1/1 -> O/1
  Fault A10/1 -> SW_1/2
  Fault A11/1 -> SW_1/5
  R-S Flip-Flop/1(Q) -> DTC_D/1
  Relational Operator4/1 -> [Arc], R-S Flip-Flop/1(S)
  R-S Flip-Flop/2(!Q) -> Terminator3/1
  DTC_B/1 -> R-S Flip-Flop/2(R)
  Ramp/1 -> Relational Operator4/2
  DTC_D/1 -> SW_1/3, SW_1/4
  [V] -> Abs3/1
  Abs3/1 -> Relational Operator4/1
  Clock/1 -> Triggered Subsystem1/1(I), Relational Operator5/1
  Triggered Subsystem1/1(O) -> Add3/1
  TimeDiff/1 -> Add3/2
  Add3/1 -> Relational Operator5/2
  SW_2/1 -> DTC_B/1
  Relational Operator5/1 -> Switch4/2
  Fault A13/1 -> Switch4/1
  Fault A14/1 -> Switch4/3
  Constant4/1 -> SW_2/2
  Demux/1 -> [I]
  Demux/2 -> [V]
  I/1 -> Demux/1
  Product/1 -> SW_2/1
  Switch4/1 -> Product/2
  Product1/1 -> Product/1, SW_2/3
  [Arc] -> Memory/1
  [I] -> Compare To Zero/1, Hit Crossing/1
  Compare To Zero/1 -> DTC_D1/1
  Hit Crossing/1 -> Product1/2
  DTC_D1/1 -> Product1/1

== system SPGF_FSK_0000_R2019b/K1/fault/Count Limiter ==
  I : Inport
  Counter : Subsystem  TreatAsAtomicUnit=on
  Fault A13 : Constant  Value=0
  Fault A3 : Constant
  Switch4 : Switch  Threshold=ArcingNumber
  Count : Outport
  O : Outport  Port=2
  wires:
  Switch4/1 -> O/1
  I/1 -> Switch4/3, Counter/Trigger
  Fault A3/1 -> Counter/1(I)
  Fault A13/1 -> Switch4/1
  Counter/1(O) -> Switch4/2, Count/1

== system SPGF_FSK_0000_R2019b/K1/fault/Fault Interruption ==
  Band-Limited White Noise1 : simulink/Sources/Band-Limited White Noise  Cov=[.1]  Ts=NoiseSampleTime  seed=NoiseSeed
  Constant1 : Constant  Value=TypeOfPause
  Fault A10 : Constant
  Fault A11 : Constant  Value=0
  Multiport Switch : MultiPortSwitch  Inputs=4  DataPortForDefault=Additional data port
  Pulse Generator : DiscretePulseGenerator  PulseType=Time based  Period=PulsePeriod  PulseWidth=PulseWidth  PhaseDelay=PhaseDelay
  Rate Transition1 : RateTransition
  Saturation1 : Saturate  UpperLimit=1  LowerLimit=0
  Sign1 : Signum
  "Stair Generator " : powerlib_meascontrol/Pulse & Signal Generators/Stair Generator  t=SwitchTimes  e=SwitchStatus  Ts=0
  O : Outport
  wires:
  Multiport Switch/1 -> O/1
  Fault A10/1 -> Multiport Switch/2
  Fault A11/1 -> Multiport Switch/6
  Sign1/1 -> Saturation1/1
  Constant1/1 -> Multiport Switch/1
  Pulse Generator/1 -> Multiport Switch/4
  Saturation1/1 -> Rate Transition1/1
  Rate Transition1/1 -> Multiport Switch/3
  "Stair Generator "/1 -> Multiport Switch/5
  Band-Limited White Noise1/1 -> Sign1/1

== system SPGF_FSK_0000_R2019b/K1/fault/Time Delay ==
  Count : Inport
  Control : Inport  Port=2
  Constant1 : Constant  Value=TimeDelay
  Constant3 : Constant  Value=0
  Memory : Memory
  SC_Time5 : Subsystem
      mask Display: disp('Delay');
  SW_Num : Switch  Threshold=ArcingNumber
  Selector : Selector  IndexMode=Zero-based  InputPortWidth=ArcingNumber  IndexOptions=Index vector (port)  Indices=[1 4]  OutputSizes=1
  O : Outport
  wires:
  SW_Num/1 -> Selector/2
  Constant3/1 -> SW_Num/1
  Selector/1 -> SC_Time5/2(TimeDelay)
  Constant1/1 -> Selector/1
  Count/1 -> Memory/1, SW_Num/2
  SC_Time5/1(Out) -> O/1
  Control/1 -> SC_Time5/1(Control)
  Memory/1 -> SW_Num/3

== system SPGF_FSK_0000_R2019b/K2/fault/Arcing ==
  I : Inport
  Enable : EnablePort  StatesWhenEnabling=reset
  Abs3 : Abs
  Add3 : Sum
  Clock : Clock
  Compare To Zero : simulink/Logic and Bit Operations/Compare To Zero  relop=~=  OutDataTypeStr=boolean
  Constant1 : Constant  Value=TheoryOfArc
  Constant4 : Constant  Value=TheoryOfArc
  DTC_B : DataTypeConversion  OutDataTypeStr=boolean
  DTC_D : DataTypeConversion  OutDataTypeStr=double
  DTC_D1 : DataTypeConversion  OutDataTypeStr=double
  Demux : Demux  Outputs=2
  Fault A10 : Constant
  Fault A11 : Constant  Value=0
  Fault A13 : Constant
  Fault A14 : Constant  Value=0
  Hit Crossing : HitCross
  Memory : Memory
  Product : Product
  Product1 : Product
  R-S Flip-Flop : Subsystem  mask(RSFlipFlop){InitialCondition=0}
      mask prompts: InitialCondition "Initial condition (state of Q)"
      mask help: R-S Flip-Flop Block
  Ramp : simulink/Sources/Ramp  slope=Slope  start=BeginFaultTime  InitialOutput=ArcingVoltage(1)
  Relational Operator4 : RelationalOperator  OutDataTypeStr=boolean  RndMeth=Nearest
  Relational Operator5 : RelationalOperator  OutDataTypeStr=boolean  RndMeth=Nearest
  SW_1 : MultiPortSwitch  DataPortForDefault=Additional data port
  SW_2 : Switch  Criteria=u2 > Threshold  Threshold=2
  Switch4 : Switch  Criteria=u2 > Threshold  Threshold=0.5
  Terminator3 : Terminator
  TimeDiff : Constant  Value=.015
  Triggered Subsystem1 : Subsystem  TreatAsAtomicUnit=on
  O : Outport  InitialOutput=[0]
  wires:
  Memory/1 -> Triggered Subsystem1/Trigger
  Constant1/1 -> SW_1/1
  SW_1/1 -> O/1
  Fault A10/1 -> SW_1/2
  Fault A11/1 -> SW_1/5
  R-S Flip-Flop/1(Q) -> DTC_D/1
  Relational Operator4/1 -> [Arc], R-S Flip-Flop/1(S)
  R-S Flip-Flop/2(!Q) -> Terminator3/1
  DTC_B/1 -> R-S Flip-Flop/2(R)
  Ramp/1 -> Relational Operator4/2
  DTC_D/1 -> SW_1/3, SW_1/4
  [V] -> Abs3/1
  Abs3/1 -> Relational Operator4/1
  Clock/1 -> Triggered Subsystem1/1(I), Relational Operator5/1
  Triggered Subsystem1/1(O) -> Add3/1
  TimeDiff/1 -> Add3/2
  Add3/1 -> Relational Operator5/2
  SW_2/1 -> DTC_B/1
  Relational Operator5/1 -> Switch4/2
  Fault A13/1 -> Switch4/1
  Fault A14/1 -> Switch4/3
  Constant4/1 -> SW_2/2
  Demux/1 -> [I]
  Demux/2 -> [V]
  I/1 -> Demux/1
  Product/1 -> SW_2/1
  Switch4/1 -> Product/2
  Product1/1 -> Product/1, SW_2/3
  [Arc] -> Memory/1
  [I] -> Compare To Zero/1, Hit Crossing/1
  Compare To Zero/1 -> DTC_D1/1
  Hit Crossing/1 -> Product1/2
  DTC_D1/1 -> Product1/1

== system SPGF_FSK_0000_R2019b/K2/fault/Count Limiter ==
  I : Inport
  Counter : Subsystem  TreatAsAtomicUnit=on
  Fault A13 : Constant  Value=0
  Fault A3 : Constant
  Switch4 : Switch  Threshold=ArcingNumber
  Count : Outport
  O : Outport  Port=2
  wires:
  Switch4/1 -> O/1
  I/1 -> Switch4/3, Counter/Trigger
  Fault A3/1 -> Counter/1(I)
  Fault A13/1 -> Switch4/1
  Counter/1(O) -> Switch4/2, Count/1

== system SPGF_FSK_0000_R2019b/K2/fault/Fault Interruption ==
  Band-Limited White Noise1 : simulink/Sources/Band-Limited White Noise  Cov=[.1]  Ts=NoiseSampleTime  seed=NoiseSeed
  Constant1 : Constant  Value=TypeOfPause
  Fault A10 : Constant
  Fault A11 : Constant  Value=0
  Multiport Switch : MultiPortSwitch  Inputs=4  DataPortForDefault=Additional data port
  Pulse Generator : DiscretePulseGenerator  PulseType=Time based  Period=PulsePeriod  PulseWidth=PulseWidth  PhaseDelay=PhaseDelay
  Rate Transition1 : RateTransition
  Saturation1 : Saturate  UpperLimit=1  LowerLimit=0
  Scope : Scope
  Sign1 : Signum
  "Stair Generator " : powerlib_meascontrol/Pulse & Signal Generators/Stair Generator  t=SwitchTimes  e=SwitchStatus  Ts=0
  Stair Generator 1 : powerlib_meascontrol/Pulse & Signal Generators/Stair Generator  t=SwitchTimes  e=SwitchStatus  Ts=0
  O : Outport
  wires:
  Stair Generator 1/1 -> Scope/1
  Multiport Switch/1 -> O/1
  Fault A10/1 -> Multiport Switch/2
  Fault A11/1 -> Multiport Switch/6
  Sign1/1 -> Saturation1/1
  Constant1/1 -> Multiport Switch/1
  Pulse Generator/1 -> Multiport Switch/4
  Saturation1/1 -> Rate Transition1/1
  Rate Transition1/1 -> Multiport Switch/3
  "Stair Generator "/1 -> Multiport Switch/5
  Band-Limited White Noise1/1 -> Sign1/1

== system SPGF_FSK_0000_R2019b/K2/fault/Time Delay ==
  Count : Inport
  Control : Inport  Port=2
  Constant1 : Constant  Value=TimeDelay
  Constant3 : Constant  Value=0
  Memory : Memory
  SC_Time5 : Subsystem
      mask Display: disp('Delay');
  SW_Num : Switch  Threshold=ArcingNumber
  Selector : Selector  IndexMode=Zero-based  InputPortWidth=ArcingNumber  IndexOptions=Index vector (port)  Indices=[1 4]  OutputSizes=1
  O : Outport
  wires:
  SW_Num/1 -> Selector/2
  Constant3/1 -> SW_Num/1
  Selector/1 -> SC_Time5/2(TimeDelay)
  Constant1/1 -> Selector/1
  Count/1 -> Memory/1, SW_Num/2
  SC_Time5/1(Out) -> O/1
  Control/1 -> SC_Time5/1(Control)
  Memory/1 -> SW_Num/3

== system SPGF_FSK_0000_R2019b/K3/fault/Arcing ==
  I : Inport
  Enable : EnablePort  StatesWhenEnabling=reset
  Abs3 : Abs
  Add3 : Sum
  Clock : Clock
  Compare To Zero : simulink/Logic and Bit Operations/Compare To Zero  relop=~=  OutDataTypeStr=boolean
  Constant1 : Constant  Value=TheoryOfArc
  Constant4 : Constant  Value=TheoryOfArc
  DTC_B : DataTypeConversion  OutDataTypeStr=boolean
  DTC_D : DataTypeConversion  OutDataTypeStr=double
  DTC_D1 : DataTypeConversion  OutDataTypeStr=double
  Demux : Demux  Outputs=2
  Fault A10 : Constant
  Fault A11 : Constant  Value=0
  Fault A13 : Constant
  Fault A14 : Constant  Value=0
  Hit Crossing : HitCross
  Memory : Memory
  Product : Product
  Product1 : Product
  R-S Flip-Flop : Subsystem  mask(RSFlipFlop){InitialCondition=0}
      mask prompts: InitialCondition "Initial condition (state of Q)"
      mask help: R-S Flip-Flop Block
  Ramp : simulink/Sources/Ramp  slope=Slope  start=BeginFaultTime  InitialOutput=ArcingVoltage(1)
  Relational Operator4 : RelationalOperator  OutDataTypeStr=boolean  RndMeth=Nearest
  Relational Operator5 : RelationalOperator  OutDataTypeStr=boolean  RndMeth=Nearest
  SW_1 : MultiPortSwitch  DataPortForDefault=Additional data port
  SW_2 : Switch  Criteria=u2 > Threshold  Threshold=2
  Scope : Scope
  Switch4 : Switch  Criteria=u2 > Threshold  Threshold=0.5
  Terminator3 : Terminator
  TimeDiff : Constant  Value=.015
  Triggered Subsystem1 : Subsystem  TreatAsAtomicUnit=on
  O : Outport  InitialOutput=[0]
  wires:
  Memory/1 -> Triggered Subsystem1/Trigger
  Constant1/1 -> SW_1/1
  SW_1/1 -> O/1
  Fault A10/1 -> SW_1/2
  Fault A11/1 -> SW_1/5
  R-S Flip-Flop/1(Q) -> DTC_D/1
  Relational Operator4/1 -> [Arc], R-S Flip-Flop/1(S)
  R-S Flip-Flop/2(!Q) -> Terminator3/1
  DTC_B/1 -> R-S Flip-Flop/2(R)
  Ramp/1 -> Relational Operator4/2
  DTC_D/1 -> SW_1/3, SW_1/4
  [V] -> Abs3/1
  Abs3/1 -> Relational Operator4/1
  Clock/1 -> Triggered Subsystem1/1(I), Relational Operator5/1
  Triggered Subsystem1/1(O) -> Add3/1
  TimeDiff/1 -> Add3/2
  Add3/1 -> Relational Operator5/2
  SW_2/1 -> DTC_B/1
  Relational Operator5/1 -> Switch4/2
  Fault A13/1 -> Switch4/1
  Fault A14/1 -> Switch4/3
  Constant4/1 -> SW_2/2
  Demux/1 -> [I]
  Demux/2 -> [V]
  I/1 -> Demux/1
  Product/1 -> SW_2/1
  Switch4/1 -> Product/2
  Product1/1 -> Scope/1, Product/1, SW_2/3
  [Arc] -> Memory/1
  [I] -> Compare To Zero/1, Hit Crossing/1
  Compare To Zero/1 -> DTC_D1/1
  Hit Crossing/1 -> Product1/2
  DTC_D1/1 -> Product1/1

== system SPGF_FSK_0000_R2019b/K3/fault/Count Limiter ==
  I : Inport
  Counter : Subsystem  TreatAsAtomicUnit=on
  Fault A13 : Constant  Value=0
  Fault A3 : Constant
  Switch4 : Switch  Threshold=ArcingNumber
  Count : Outport
  O : Outport  Port=2
  wires:
  Switch4/1 -> O/1
  I/1 -> Switch4/3, Counter/Trigger
  Fault A3/1 -> Counter/1(I)
  Fault A13/1 -> Switch4/1
  Counter/1(O) -> Switch4/2, Count/1
